simulink model "CM475A_TSG31CfgAndUse"  (R2013b)
settings: Solver=FixedStepDiscrete  SolverMode=SingleTasking  StartTime=0.0  StopTime=0.01  FixedStep=0.00005  RelTol=1e-3
values from neighbouring files (symbols this model uses):
  ELECGLBPRM_MOTCTRLINTRPTTRIGCFGB_CNT_U08 = DataDict.Constant    [CM475A_TSG31CfgAndUse_DataDict.m]
  ELECGLBPRM_MOTCTRLINTRPTTRIGSRC_CNT_U08 = DataDict.ConfigParam    [CM475A_TSG31CfgAndUse_DataDict.m]
  ELECGLBPRM_PWMPERDMIN_NANOSEC_U32 = DataDict.ConfigParam    [CM475A_TSG31CfgAndUse_DataDict.m]
  TSG31CfgAndUseAdcStrtOfCnvn2Offs = DataDict.Calibration    [CM475A_TSG31CfgAndUse_DataDict.m]
  TSG31CfgAndUseAdcStrtOfCnvnMotCtrlPeakOffs = DataDict.Calibration    [CM475A_TSG31CfgAndUse_DataDict.m]
  TSG31CfgAndUseAdcStrtOfCnvnMotCtrlVlyOffs = DataDict.Calibration    [CM475A_TSG31CfgAndUse_DataDict.m]
  TSG31CfgAndUseMtrAg0SPIStart = DataDict.Calibration    [CM475A_TSG31CfgAndUse_DataDict.m]
  TSG31CfgAndUsePwmDbnd = DataDict.Calibration    [CM475A_TSG31CfgAndUse_DataDict.m]
  TSG31UPD_NANOSEC_U32 = DataDict.Constant    [CM475A_TSG31CfgAndUse_DataDict.m]
undefined symbols (not defined in the file or in its folder): sigbuilder_block, SysSt1
libraries: simulink x11, CM475A_TSG31CfgAndUse_ModelLibrary_Rev001 x11
(part 3 of 5)

== system CM475A_TSG31CfgAndUse/TSG31CfgAndUse/TSG31CfgAndUsePer2/Transition to Enable/Map Pins to Peripheral/IoHwAb_SetFctPeriphPhaBLowrCmd ==
  CopyRight2 : Subsystem  Description=|  mask(Copyright Information){none=on}
      | Copyright info block.                                               
      |                                                                     
      | Place copyright information at the top of every subsystem in design.
      mask prompts: none "No parameters"
      mask help: Place copyright information at the top of every subsystem in design.
      mask Display:
      | NxtrConf = 'Nexteer Confidential';
      | 
      | sys = bdroot; %handle for the current model ("system")
      | first = get_param(sys,'Created');
      | first = first(end-3:end);  %year is last four digits
      | 
      | last = get_param(sys,'LastModifiedDate');
      | if isempty(last)
      |     last = datestr(now,'yyyy');
      | else
      |     last = last(end-3:end);
      | end
      | 
      | if strcmp(first,last)
      |     fprintf('%s -- Copyright %s Nexteer',NxtrConf,first)
      | else
      |     fprintf('%s -- %s%s- %s Nexteer',NxtrConf,char(169),first,last)
      | end

== system CM475A_TSG31CfgAndUse/TSG31CfgAndUse/TSG31CfgAndUsePer2/Transition to Enable/Map Pins to Peripheral/IoHwAb_SetFctPeriphPhaBUpprCmd ==
  CopyRight2 : Subsystem  Description=|  mask(Copyright Information){none=on}
      | Copyright info block.                                               
      |                                                                     
      | Place copyright information at the top of every subsystem in design.
      mask prompts: none "No parameters"
      mask help: Place copyright information at the top of every subsystem in design.
      mask Display:
      | NxtrConf = 'Nexteer Confidential';
      | 
      | sys = bdroot; %handle for the current model ("system")
      | first = get_param(sys,'Created');
      | first = first(end-3:end);  %year is last four digits
      | 
      | last = get_param(sys,'LastModifiedDate');
      | if isempty(last)
      |     last = datestr(now,'yyyy');
      | else
      |     last = last(end-3:end);
      | end
      | 
      | if strcmp(first,last)
      |     fprintf('%s -- Copyright %s Nexteer',NxtrConf,first)
      | else
      |     fprintf('%s -- %s%s- %s Nexteer',NxtrConf,char(169),first,last)
      | end

== system CM475A_TSG31CfgAndUse/TSG31CfgAndUse/TSG31CfgAndUsePer2/Transition to Enable/Map Pins to Peripheral/IoHwAb_SetFctPeriphPhaCLowrCmd ==
  CopyRight2 : Subsystem  Description=|  mask(Copyright Information){none=on}
      | Copyright info block.                                               
      |                                                                     
      | Place copyright information at the top of every subsystem in design.
      mask prompts: none "No parameters"
      mask help: Place copyright information at the top of every subsystem in design.
      mask Display:
      | NxtrConf = 'Nexteer Confidential';
      | 
      | sys = bdroot; %handle for the current model ("system")
      | first = get_param(sys,'Created');
      | first = first(end-3:end);  %year is last four digits
      | 
      | last = get_param(sys,'LastModifiedDate');
      | if isempty(last)
      |     last = datestr(now,'yyyy');
      | else
      |     last = last(end-3:end);
      | end
      | 
      | if strcmp(first,last)
      |     fprintf('%s -- Copyright %s Nexteer',NxtrConf,first)
      | else
      |     fprintf('%s -- %s%s- %s Nexteer',NxtrConf,char(169),first,last)
      | end

== system CM475A_TSG31CfgAndUse/TSG31CfgAndUse/TSG31CfgAndUsePer2/Transition to Enable/Map Pins to Peripheral/IoHwAb_SetFctPeriphPhaCUpprCmd ==
  CopyRight2 : Subsystem  Description=|  mask(Copyright Information){none=on}
      | Copyright info block.                                               
      |                                                                     
      | Place copyright information at the top of every subsystem in design.
      mask prompts: none "No parameters"
      mask help: Place copyright information at the top of every subsystem in design.
      mask Display:
      | NxtrConf = 'Nexteer Confidential';
      | 
      | sys = bdroot; %handle for the current model ("system")
      | first = get_param(sys,'Created');
      | first = first(end-3:end);  %year is last four digits
      | 
      | last = get_param(sys,'LastModifiedDate');
      | if isempty(last)
      |     last = datestr(now,'yyyy');
      | else
      |     last = last(end-3:end);
      | end
      | 
      | if strcmp(first,last)
      |     fprintf('%s -- Copyright %s Nexteer',NxtrConf,first)
      | else
      |     fprintf('%s -- %s%s- %s Nexteer',NxtrConf,char(169),first,last)
      | end

== system CM475A_TSG31CfgAndUse/TSG31CfgAndUse/TSG31CfgAndUseInit1/Determine TSG31CTL4/Determine TSG31PIE/Config - B/CopyRight2 ==

== system CM475A_TSG31CfgAndUse/TSG31CfgAndUse/TSG31CfgAndUseInit1/Determine TSG31CTL4/Determine TSG31PIE/Default Config/CopyRight2 ==

== system CM475A_TSG31CfgAndUse/TSG31CfgAndUse/TSG31CfgAndUseInit1/Map FET Ctrl Signals to GPIO and Set Low/Map Pins to GPIO/IoHwAb_SetFctGpioPhaALowrCmd/CopyRight2 ==

== system CM475A_TSG31CfgAndUse/TSG31CfgAndUse/TSG31CfgAndUseInit1/Map FET Ctrl Signals to GPIO and Set Low/Map Pins to GPIO/IoHwAb_SetFctGpioPhaAUpprCmd/CopyRight2 ==

== system CM475A_TSG31CfgAndUse/TSG31CfgAndUse/TSG31CfgAndUseInit1/Map FET Ctrl Signals to GPIO and Set Low/Map Pins to GPIO/IoHwAb_SetFctGpioPhaBLowrCmd/CopyRight2 ==

== system CM475A_TSG31CfgAndUse/TSG31CfgAndUse/TSG31CfgAndUseInit1/Map FET Ctrl Signals to GPIO and Set Low/Map Pins to GPIO/IoHwAb_SetFctGpioPhaBUpprCmd/CopyRight2 ==

== system CM475A_TSG31CfgAndUse/TSG31CfgAndUse/TSG31CfgAndUseInit1/Map FET Ctrl Signals to GPIO and Set Low/Map Pins to GPIO/IoHwAb_SetFctGpioPhaCLowrCmd/CopyRight2 ==

== system CM475A_TSG31CfgAndUse/TSG31CfgAndUse/TSG31CfgAndUseInit1/Map FET Ctrl Signals to GPIO and Set Low/Map Pins to GPIO/IoHwAb_SetFctGpioPhaCUpprCmd/CopyRight2 ==

== system CM475A_TSG31CfgAndUse/TSG31CfgAndUse/TSG31CfgAndUseInit1/Map FET Ctrl Signals to GPIO and Set Low/Set GPIO Level/IoHwAb_SetGpioPhaALowrCmd/CopyRight2 ==

== system CM475A_TSG31CfgAndUse/TSG31CfgAndUse/TSG31CfgAndUseInit1/Map FET Ctrl Signals to GPIO and Set Low/Set GPIO Level/IoHwAb_SetGpioPhaAUpprCmd/CopyRight2 ==

== system CM475A_TSG31CfgAndUse/TSG31CfgAndUse/TSG31CfgAndUseInit1/Map FET Ctrl Signals to GPIO and Set Low/Set GPIO Level/IoHwAb_SetGpioPhaBLowrCmd/CopyRight2 ==

== system CM475A_TSG31CfgAndUse/TSG31CfgAndUse/TSG31CfgAndUseInit1/Map FET Ctrl Signals to GPIO and Set Low/Set GPIO Level/IoHwAb_SetGpioPhaBUpprCmd/CopyRight2 ==

== system CM475A_TSG31CfgAndUse/TSG31CfgAndUse/TSG31CfgAndUseInit1/Map FET Ctrl Signals to GPIO and Set Low/Set GPIO Level/IoHwAb_SetGpioPhaCLowrCmd/CopyRight2 ==

== system CM475A_TSG31CfgAndUse/TSG31CfgAndUse/TSG31CfgAndUseInit1/Map FET Ctrl Signals to GPIO and Set Low/Set GPIO Level/IoHwAb_SetGpioPhaCUpprCmd/CopyRight2 ==

== system CM475A_TSG31CfgAndUse/TSG31CfgAndUse/TSG31CfgAndUsePer2/No Transition SysState = Enable/MCECS_CMDSAFEST/Map Pins to GPIO/CopyRight2 ==

== system CM475A_TSG31CfgAndUse/TSG31CfgAndUse/TSG31CfgAndUsePer2/No Transition SysState = Enable/MCECS_CMDSAFEST/Map Pins to GPIO/IoHwAb_SetFctGpioPhaALowrCmd ==
  CopyRight2 : Subsystem  Description=|  mask(Copyright Information){none=on}
      | Copyright info block.                                               
      |                                                                     
      | Place copyright information at the top of every subsystem in design.
      mask prompts: none "No parameters"
      mask help: Place copyright information at the top of every subsystem in design.
      mask Display:
      | NxtrConf = 'Nexteer Confidential';
      | 
      | sys = bdroot; %handle for the current model ("system")
      | first = get_param(sys,'Created');
      | first = first(end-3:end);  %year is last four digits
      | 
      | last = get_param(sys,'LastModifiedDate');
      | if isempty(last)
      |     last = datestr(now,'yyyy');
      | else
      |     last = last(end-3:end);
      | end
      | 
      | if strcmp(first,last)
      |     fprintf('%s -- Copyright %s Nexteer',NxtrConf,first)
      | else
      |     fprintf('%s -- %s%s- %s Nexteer',NxtrConf,char(169),first,last)
      | end

== system CM475A_TSG31CfgAndUse/TSG31CfgAndUse/TSG31CfgAndUsePer2/No Transition SysState = Enable/MCECS_CMDSAFEST/Map Pins to GPIO/IoHwAb_SetFctGpioPhaAUpprCmd ==
  CopyRight2 : Subsystem  Description=|  mask(Copyright Information){none=on}
      | Copyright info block.                                               
      |                                                                     
      | Place copyright information at the top of every subsystem in design.
      mask prompts: none "No parameters"
      mask help: Place copyright information at the top of every subsystem in design.
      mask Display:
      | NxtrConf = 'Nexteer Confidential';
      | 
      | sys = bdroot; %handle for the current model ("system")
      | first = get_param(sys,'Created');
      | first = first(end-3:end);  %year is last four digits
      | 
      | last = get_param(sys,'LastModifiedDate');
      | if isempty(last)
      |     last = datestr(now,'yyyy');
      | else
      |     last = last(end-3:end);
      | end
      | 
      | if strcmp(first,last)
      |     fprintf('%s -- Copyright %s Nexteer',NxtrConf,first)
      | else
      |     fprintf('%s -- %s%s- %s Nexteer',NxtrConf,char(169),first,last)
      | end

== system CM475A_TSG31CfgAndUse/TSG31CfgAndUse/TSG31CfgAndUsePer2/No Transition SysState = Enable/MCECS_CMDSAFEST/Map Pins to GPIO/IoHwAb_SetFctGpioPhaBLowrCmd ==
  CopyRight2 : Subsystem  Description=|  mask(Copyright Information){none=on}
      | Copyright info block.                                               
      |                                                                     
      | Place copyright information at the top of every subsystem in design.
      mask prompts: none "No parameters"
      mask help: Place copyright information at the top of every subsystem in design.
      mask Display:
      | NxtrConf = 'Nexteer Confidential';
      | 
      | sys = bdroot; %handle for the current model ("system")
      | first = get_param(sys,'Created');
      | first = first(end-3:end);  %year is last four digits
      | 
      | last = get_param(sys,'LastModifiedDate');
      | if isempty(last)
      |     last = datestr(now,'yyyy');
      | else
      |     last = last(end-3:end);
      | end
      | 
      | if strcmp(first,last)
      |     fprintf('%s -- Copyright %s Nexteer',NxtrConf,first)
      | else
      |     fprintf('%s -- %s%s- %s Nexteer',NxtrConf,char(169),first,last)
      | end

== system CM475A_TSG31CfgAndUse/TSG31CfgAndUse/TSG31CfgAndUsePer2/No Transition SysState = Enable/MCECS_CMDSAFEST/Map Pins to GPIO/IoHwAb_SetFctGpioPhaBUpprCmd ==
  CopyRight2 : Subsystem  Description=|  mask(Copyright Information){none=on}
      | Copyright info block.                                               
      |                                                                     
      | Place copyright information at the top of every subsystem in design.
      mask prompts: none "No parameters"
      mask help: Place copyright information at the top of every subsystem in design.
      mask Display:
      | NxtrConf = 'Nexteer Confidential';
      | 
      | sys = bdroot; %handle for the current model ("system")
      | first = get_param(sys,'Created');
      | first = first(end-3:end);  %year is last four digits
      | 
      | last = get_param(sys,'LastModifiedDate');
      | if isempty(last)
      |     last = datestr(now,'yyyy');
      | else
      |     last = last(end-3:end);
      | end
      | 
      | if strcmp(first,last)
      |     fprintf('%s -- Copyright %s Nexteer',NxtrConf,first)
      | else
      |     fprintf('%s -- %s%s- %s Nexteer',NxtrConf,char(169),first,last)
      | end

== system CM475A_TSG31CfgAndUse/TSG31CfgAndUse/TSG31CfgAndUsePer2/No Transition SysState = Enable/MCECS_CMDSAFEST/Map Pins to GPIO/IoHwAb_SetFctGpioPhaCLowrCmd ==
  CopyRight2 : Subsystem  Description=|  mask(Copyright Information){none=on}
      | Copyright info block.                                               
      |                                                                     
      | Place copyright information at the top of every subsystem in design.
      mask prompts: none "No parameters"
      mask help: Place copyright information at the top of every subsystem in design.
      mask Display:
      | NxtrConf = 'Nexteer Confidential';
      | 
      | sys = bdroot; %handle for the current model ("system")
      | first = get_param(sys,'Created');
      | first = first(end-3:end);  %year is last four digits
      | 
      | last = get_param(sys,'LastModifiedDate');
      | if isempty(last)
      |     last = datestr(now,'yyyy');
      | else
      |     last = last(end-3:end);
      | end
      | 
      | if strcmp(first,last)
      |     fprintf('%s -- Copyright %s Nexteer',NxtrConf,first)
      | else
      |     fprintf('%s -- %s%s- %s Nexteer',NxtrConf,char(169),first,last)
      | end

== system CM475A_TSG31CfgAndUse/TSG31CfgAndUse/TSG31CfgAndUsePer2/No Transition SysState = Enable/MCECS_CMDSAFEST/Map Pins to GPIO/IoHwAb_SetFctGpioPhaCUpprCmd ==
  CopyRight2 : Subsystem  Description=|  mask(Copyright Information){none=on}
      | Copyright info block.                                               
      |                                                                     
      | Place copyright information at the top of every subsystem in design.
      mask prompts: none "No parameters"
      mask help: Place copyright information at the top of every subsystem in design.
      mask Display:
      | NxtrConf = 'Nexteer Confidential';
      | 
      | sys = bdroot; %handle for the current model ("system")
      | first = get_param(sys,'Created');
      | first = first(end-3:end);  %year is last four digits
      | 
      | last = get_param(sys,'LastModifiedDate');
      | if isempty(last)
      |     last = datestr(now,'yyyy');
      | else
      |     last = last(end-3:end);
      | end
      | 
      | if strcmp(first,last)
      |     fprintf('%s -- Copyright %s Nexteer',NxtrConf,first)
      | else
      |     fprintf('%s -- %s%s- %s Nexteer',NxtrConf,char(169),first,last)
      | end

== system CM475A_TSG31CfgAndUse/TSG31CfgAndUse/TSG31CfgAndUsePer2/No Transition SysState = Enable/MCECS_CMDSAFEST/Set GPIO Level/CopyRight2 ==

== system CM475A_TSG31CfgAndUse/TSG31CfgAndUse/TSG31CfgAndUsePer2/No Transition SysState = Enable/MCECS_CMDSAFEST/Set GPIO Level/IoHwAb_SetGpioPhaALowrCmd ==
  PinSt : Inport  OutDataTypeStr=boolean
  CopyRight2 : Subsystem  Description=|  mask(Copyright Information){none=on}
      | Copyright info block.                                               
      |                                                                     
      | Place copyright information at the top of every subsystem in design.
      mask prompts: none "No parameters"
      mask help: Place copyright information at the top of every subsystem in design.
      mask Display:
      | NxtrConf = 'Nexteer Confidential';
      | 
      | sys = bdroot; %handle for the current model ("system")
      | first = get_param(sys,'Created');
      | first = first(end-3:end);  %year is last four digits
      | 
      | last = get_param(sys,'LastModifiedDate');
      | if isempty(last)
      |     last = datestr(now,'yyyy');
      | else
      |     last = last(end-3:end);
      | end
      | 
      | if strcmp(first,last)
      |     fprintf('%s -- Copyright %s Nexteer',NxtrConf,first)
      | else
      |     fprintf('%s -- %s%s- %s Nexteer',NxtrConf,char(169),first,last)
      | end
  Terminator : Terminator
  wires:
  PinSt/1 -> Terminator/1

== system CM475A_TSG31CfgAndUse/TSG31CfgAndUse/TSG31CfgAndUsePer2/No Transition SysState = Enable/MCECS_CMDSAFEST/Set GPIO Level/IoHwAb_SetGpioPhaAUpprCmd ==
  PinSt : Inport  OutDataTypeStr=boolean
  CopyRight2 : Subsystem  Description=|  mask(Copyright Information){none=on}
      | Copyright info block.                                               
      |                                                                     
      | Place copyright information at the top of every subsystem in design.
      mask prompts: none "No parameters"
      mask help: Place copyright information at the top of every subsystem in design.
      mask Display:
      | NxtrConf = 'Nexteer Confidential';
      | 
      | sys = bdroot; %handle for the current model ("system")
      | first = get_param(sys,'Created');
      | first = first(end-3:end);  %year is last four digits
      | 
      | last = get_param(sys,'LastModifiedDate');
      | if isempty(last)
      |     last = datestr(now,'yyyy');
      | else
      |     last = last(end-3:end);
      | end
      | 
      | if strcmp(first,last)
      |     fprintf('%s -- Copyright %s Nexteer',NxtrConf,first)
      | else
      |     fprintf('%s -- %s%s- %s Nexteer',NxtrConf,char(169),first,last)
      | end
  Terminator : Terminator
  wires:
  PinSt/1 -> Terminator/1

== system CM475A_TSG31CfgAndUse/TSG31CfgAndUse/TSG31CfgAndUsePer2/No Transition SysState = Enable/MCECS_CMDSAFEST/Set GPIO Level/IoHwAb_SetGpioPhaBLowrCmd ==
  PinSt : Inport  OutDataTypeStr=boolean
  CopyRight2 : Subsystem  Description=|  mask(Copyright Information){none=on}
      | Copyright info block.                                               
      |                                                                     
      | Place copyright information at the top of every subsystem in design.
      mask prompts: none "No parameters"
      mask help: Place copyright information at the top of every subsystem in design.
      mask Display:
      | NxtrConf = 'Nexteer Confidential';
      | 
      | sys = bdroot; %handle for the current model ("system")
      | first = get_param(sys,'Created');
      | first = first(end-3:end);  %year is last four digits
      | 
      | last = get_param(sys,'LastModifiedDate');
      | if isempty(last)
      |     last = datestr(now,'yyyy');
      | else
      |     last = last(end-3:end);
      | end
      | 
      | if strcmp(first,last)
      |     fprintf('%s -- Copyright %s Nexteer',NxtrConf,first)
      | else
      |     fprintf('%s -- %s%s- %s Nexteer',NxtrConf,char(169),first,last)
      | end
  Terminator : Terminator
  wires:
  PinSt/1 -> Terminator/1

== system CM475A_TSG31CfgAndUse/TSG31CfgAndUse/TSG31CfgAndUsePer2/No Transition SysState = Enable/MCECS_CMDSAFEST/Set GPIO Level/IoHwAb_SetGpioPhaBUpprCmd ==
  PinSt : Inport  OutDataTypeStr=boolean
  CopyRight2 : Subsystem  Description=|  mask(Copyright Information){none=on}
      | Copyright info block.                                               
      |                                                                     
      | Place copyright information at the top of every subsystem in design.
      mask prompts: none "No parameters"
      mask help: Place copyright information at the top of every subsystem in design.
      mask Display:
      | NxtrConf = 'Nexteer Confidential';
      | 
      | sys = bdroot; %handle for the current model ("system")
      | first = get_param(sys,'Created');
      | first = first(end-3:end);  %year is last four digits
      | 
      | last = get_param(sys,'LastModifiedDate');
      | if isempty(last)
      |     last = datestr(now,'yyyy');
      | else
      |     last = last(end-3:end);
      | end
      | 
      | if strcmp(first,last)
      |     fprintf('%s -- Copyright %s Nexteer',NxtrConf,first)
      | else
      |     fprintf('%s -- %s%s- %s Nexteer',NxtrConf,char(169),first,last)
      | end
  Terminator : Terminator
  wires:
  PinSt/1 -> Terminator/1

== system CM475A_TSG31CfgAndUse/TSG31CfgAndUse/TSG31CfgAndUsePer2/No Transition SysState = Enable/MCECS_CMDSAFEST/Set GPIO Level/IoHwAb_SetGpioPhaCLowrCmd ==
  PinSt : Inport  OutDataTypeStr=boolean
  CopyRight2 : Subsystem  Description=|  mask(Copyright Information){none=on}
      | Copyright info block.                                               
      |                                                                     
      | Place copyright information at the top of every subsystem in design.
      mask prompts: none "No parameters"
      mask help: Place copyright information at the top of every subsystem in design.
      mask Display:
      | NxtrConf = 'Nexteer Confidential';
      | 
      | sys = bdroot; %handle for the current model ("system")
      | first = get_param(sys,'Created');
      | first = first(end-3:end);  %year is last four digits
      | 
      | last = get_param(sys,'LastModifiedDate');
      | if isempty(last)
      |     last = datestr(now,'yyyy');
      | else
      |     last = last(end-3:end);
      | end
      | 
      | if strcmp(first,last)
      |     fprintf('%s -- Copyright %s Nexteer',NxtrConf,first)
      | else
      |     fprintf('%s -- %s%s- %s Nexteer',NxtrConf,char(169),first,last)
      | end
  Terminator : Terminator
  wires:
  PinSt/1 -> Terminator/1

== system CM475A_TSG31CfgAndUse/TSG31CfgAndUse/TSG31CfgAndUsePer2/No Transition SysState = Enable/MCECS_CMDSAFEST/Set GPIO Level/IoHwAb_SetGpioPhaCUpprCmd ==
  PinSt : Inport  OutDataTypeStr=boolean
  CopyRight2 : Subsystem  Description=|  mask(Copyright Information){none=on}
      | Copyright info block.                                               
      |                                                                     
      | Place copyright information at the top of every subsystem in design.
      mask prompts: none "No parameters"
      mask help: Place copyright information at the top of every subsystem in design.
      mask Display:
      | NxtrConf = 'Nexteer Confidential';
      | 
      | sys = bdroot; %handle for the current model ("system")
      | first = get_param(sys,'Created');
      | first = first(end-3:end);  %year is last four digits
      | 
      | last = get_param(sys,'LastModifiedDate');
      | if isempty(last)
      |     last = datestr(now,'yyyy');
      | else
      |     last = last(end-3:end);
      | end
      | 
      | if strcmp(first,last)
      |     fprintf('%s -- Copyright %s Nexteer',NxtrConf,first)
      | else
      |     fprintf('%s -- %s%s- %s Nexteer',NxtrConf,char(169),first,last)
      | end
  Terminator : Terminator
  wires:
  PinSt/1 -> Terminator/1

== system CM475A_TSG31CfgAndUse/TSG31CfgAndUse/TSG31CfgAndUsePer2/No Transition SysState = Enable/MCECS_GAINCMDBE/Map Pins to GPIO/CopyRight2 ==

== system CM475A_TSG31CfgAndUse/TSG31CfgAndUse/TSG31CfgAndUsePer2/No Transition SysState = Enable/MCECS_GAINCMDBE/Map Pins to GPIO/IoHwAb_SetFctGpioPhaALowrCmd ==
  CopyRight2 : Subsystem  Description=|  mask(Copyright Information){none=on}
      | Copyright info block.                                               
      |                                                                     
      | Place copyright information at the top of every subsystem in design.
      mask prompts: none "No parameters"
      mask help: Place copyright information at the top of every subsystem in design.
      mask Display:
      | NxtrConf = 'Nexteer Confidential';
      | 
      | sys = bdroot; %handle for the current model ("system")
      | first = get_param(sys,'Created');
      | first = first(end-3:end);  %year is last four digits
      | 
      | last = get_param(sys,'LastModifiedDate');
      | if isempty(last)
      |     last = datestr(now,'yyyy');
      | else
      |     last = last(end-3:end);
      | end
      | 
      | if strcmp(first,last)
      |     fprintf('%s -- Copyright %s Nexteer',NxtrConf,first)
      | else
      |     fprintf('%s -- %s%s- %s Nexteer',NxtrConf,char(169),first,last)
      | end

== system CM475A_TSG31CfgAndUse/TSG31CfgAndUse/TSG31CfgAndUsePer2/No Transition SysState = Enable/MCECS_GAINCMDBE/Map Pins to GPIO/IoHwAb_SetFctGpioPhaAUpprCmd ==
  CopyRight2 : Subsystem  Description=|  mask(Copyright Information){none=on}
      | Copyright info block.                                               
      |                                                                     
      | Place copyright information at the top of every subsystem in design.
      mask prompts: none "No parameters"
      mask help: Place copyright information at the top of every subsystem in design.
      mask Display:
      | NxtrConf = 'Nexteer Confidential';
      | 
      | sys = bdroot; %handle for the current model ("system")
      | first = get_param(sys,'Created');
      | first = first(end-3:end);  %year is last four digits
      | 
      | last = get_param(sys,'LastModifiedDate');
      | if isempty(last)
      |     last = datestr(now,'yyyy');
      | else
      |     last = last(end-3:end);
      | end
      | 
      | if strcmp(first,last)
      |     fprintf('%s -- Copyright %s Nexteer',NxtrConf,first)
      | else
      |     fprintf('%s -- %s%s- %s Nexteer',NxtrConf,char(169),first,last)
      | end

== system CM475A_TSG31CfgAndUse/TSG31CfgAndUse/TSG31CfgAndUsePer2/No Transition SysState = Enable/MCECS_GAINCMDBE/Map Pins to GPIO/IoHwAb_SetFctGpioPhaBLowrCmd ==
  CopyRight2 : Subsystem  Description=|  mask(Copyright Information){none=on}
      | Copyright info block.                                               
      |                                                                     
      | Place copyright information at the top of every subsystem in design.
      mask prompts: none "No parameters"
      mask help: Place copyright information at the top of every subsystem in design.
      mask Display:
      | NxtrConf = 'Nexteer Confidential';
      | 
      | sys = bdroot; %handle for the current model ("system")
      | first = get_param(sys,'Created');
      | first = first(end-3:end);  %year is last four digits
      | 
      | last = get_param(sys,'LastModifiedDate');
      | if isempty(last)
      |     last = datestr(now,'yyyy');
      | else
      |     last = last(end-3:end);
      | end
      | 
      | if strcmp(first,last)
      |     fprintf('%s -- Copyright %s Nexteer',NxtrConf,first)
      | else
      |     fprintf('%s -- %s%s- %s Nexteer',NxtrConf,char(169),first,last)
      | end

== system CM475A_TSG31CfgAndUse/TSG31CfgAndUse/TSG31CfgAndUsePer2/No Transition SysState = Enable/MCECS_GAINCMDBE/Map Pins to GPIO/IoHwAb_SetFctGpioPhaBUpprCmd ==
  CopyRight2 : Subsystem  Description=|  mask(Copyright Information){none=on}
      | Copyright info block.                                               
      |                                                                     
      | Place copyright information at the top of every subsystem in design.
      mask prompts: none "No parameters"
      mask help: Place copyright information at the top of every subsystem in design.
      mask Display:
      | NxtrConf = 'Nexteer Confidential';
      | 
      | sys = bdroot; %handle for the current model ("system")
      | first = get_param(sys,'Created');
      | first = first(end-3:end);  %year is last four digits
      | 
      | last = get_param(sys,'LastModifiedDate');
      | if isempty(last)
      |     last = datestr(now,'yyyy');
      | else
      |     last = last(end-3:end);
      | end
      | 
      | if strcmp(first,last)
      |     fprintf('%s -- Copyright %s Nexteer',NxtrConf,first)
      | else
      |     fprintf('%s -- %s%s- %s Nexteer',NxtrConf,char(169),first,last)
      | end

== system CM475A_TSG31CfgAndUse/TSG31CfgAndUse/TSG31CfgAndUsePer2/No Transition SysState = Enable/MCECS_GAINCMDBE/Map Pins to GPIO/IoHwAb_SetFctGpioPhaCLowrCmd ==
  CopyRight2 : Subsystem  Description=|  mask(Copyright Information){none=on}
      | Copyright info block.                                               
      |                                                                     
      | Place copyright information at the top of every subsystem in design.
      mask prompts: none "No parameters"
      mask help: Place copyright information at the top of every subsystem in design.
      mask Display:
      | NxtrConf = 'Nexteer Confidential';
      | 
      | sys = bdroot; %handle for the current model ("system")
      | first = get_param(sys,'Created');
      | first = first(end-3:end);  %year is last four digits
      | 
      | last = get_param(sys,'LastModifiedDate');
      | if isempty(last)
      |     last = datestr(now,'yyyy');
      | else
      |     last = last(end-3:end);
      | end
      | 
      | if strcmp(first,last)
      |     fprintf('%s -- Copyright %s Nexteer',NxtrConf,first)
      | else
      |     fprintf('%s -- %s%s- %s Nexteer',NxtrConf,char(169),first,last)
      | end

== system CM475A_TSG31CfgAndUse/TSG31CfgAndUse/TSG31CfgAndUsePer2/No Transition SysState = Enable/MCECS_GAINCMDBE/Map Pins to GPIO/IoHwAb_SetFctGpioPhaCUpprCmd ==
  CopyRight2 : Subsystem  Description=|  mask(Copyright Information){none=on}
      | Copyright info block.                                               
      |                                                                     
      | Place copyright information at the top of every subsystem in design.
      mask prompts: none "No parameters"
      mask help: Place copyright information at the top of every subsystem in design.
      mask Display:
      | NxtrConf = 'Nexteer Confidential';
      | 
      | sys = bdroot; %handle for the current model ("system")
      | first = get_param(sys,'Created');
      | first = first(end-3:end);  %year is last four digits
      | 
      | last = get_param(sys,'LastModifiedDate');
      | if isempty(last)
      |     last = datestr(now,'yyyy');
      | else
      |     last = last(end-3:end);
      | end
      | 
      | if strcmp(first,last)
      |     fprintf('%s -- Copyright %s Nexteer',NxtrConf,first)
      | else
      |     fprintf('%s -- %s%s- %s Nexteer',NxtrConf,char(169),first,last)
      | end

== system CM475A_TSG31CfgAndUse/TSG31CfgAndUse/TSG31CfgAndUsePer2/No Transition SysState = Enable/MCECS_GAINCMDBE/Set GPIO Level/CopyRight2 ==

== system CM475A_TSG31CfgAndUse/TSG31CfgAndUse/TSG31CfgAndUsePer2/No Transition SysState = Enable/MCECS_GAINCMDBE/Set GPIO Level/IoHwAb_SetGpioPhaALowrCmd ==
  PinSt : Inport  OutDataTypeStr=boolean
  CopyRight2 : Subsystem  Description=|  mask(Copyright Information){none=on}
      | Copyright info block.                                               
      |                                                                     
      | Place copyright information at the top of every subsystem in design.
      mask prompts: none "No parameters"
      mask help: Place copyright information at the top of every subsystem in design.
      mask Display:
      | NxtrConf = 'Nexteer Confidential';
      | 
      | sys = bdroot; %handle for the current model ("system")
      | first = get_param(sys,'Created');
      | first = first(end-3:end);  %year is last four digits
      | 
      | last = get_param(sys,'LastModifiedDate');
      | if isempty(last)
      |     last = datestr(now,'yyyy');
      | else
      |     last = last(end-3:end);
      | end
      | 
      | if strcmp(first,last)
      |     fprintf('%s -- Copyright %s Nexteer',NxtrConf,first)
      | else
      |     fprintf('%s -- %s%s- %s Nexteer',NxtrConf,char(169),first,last)
      | end
  Terminator : Terminator
  wires:
  PinSt/1 -> Terminator/1

== system CM475A_TSG31CfgAndUse/TSG31CfgAndUse/TSG31CfgAndUsePer2/No Transition SysState = Enable/MCECS_GAINCMDBE/Set GPIO Level/IoHwAb_SetGpioPhaAUpprCmd ==
  PinSt : Inport  OutDataTypeStr=boolean
  CopyRight2 : Subsystem  Description=|  mask(Copyright Information){none=on}
      | Copyright info block.                                               
      |                                                                     
      | Place copyright information at the top of every subsystem in design.
      mask prompts: none "No parameters"
      mask help: Place copyright information at the top of every subsystem in design.
      mask Display:
      | NxtrConf = 'Nexteer Confidential';
      | 
      | sys = bdroot; %handle for the current model ("system")
      | first = get_param(sys,'Created');
      | first = first(end-3:end);  %year is last four digits
      | 
      | last = get_param(sys,'LastModifiedDate');
      | if isempty(last)
      |     last = datestr(now,'yyyy');
      | else
      |     last = last(end-3:end);
      | end
      | 
      | if strcmp(first,last)
      |     fprintf('%s -- Copyright %s Nexteer',NxtrConf,first)
      | else
      |     fprintf('%s -- %s%s- %s Nexteer',NxtrConf,char(169),first,last)
      | end
  Terminator : Terminator
  wires:
  PinSt/1 -> Terminator/1

== system CM475A_TSG31CfgAndUse/TSG31CfgAndUse/TSG31CfgAndUsePer2/No Transition SysState = Enable/MCECS_GAINCMDBE/Set GPIO Level/IoHwAb_SetGpioPhaBLowrCmd ==
  PinSt : Inport  OutDataTypeStr=boolean
  CopyRight2 : Subsystem  Description=|  mask(Copyright Information){none=on}
      | Copyright info block.                                               
      |                                                                     
      | Place copyright information at the top of every subsystem in design.
      mask prompts: none "No parameters"
      mask help: Place copyright information at the top of every subsystem in design.
      mask Display:
      | NxtrConf = 'Nexteer Confidential';
      | 
      | sys = bdroot; %handle for the current model ("system")
      | first = get_param(sys,'Created');
      | first = first(end-3:end);  %year is last four digits
      | 
      | last = get_param(sys,'LastModifiedDate');
      | if isempty(last)
      |     last = datestr(now,'yyyy');
      | else
      |     last = last(end-3:end);
      | end
      | 
      | if strcmp(first,last)
      |     fprintf('%s -- Copyright %s Nexteer',NxtrConf,first)
      | else
      |     fprintf('%s -- %s%s- %s Nexteer',NxtrConf,char(169),first,last)
      | end
  Terminator : Terminator
  wires:
  PinSt/1 -> Terminator/1

== system CM475A_TSG31CfgAndUse/TSG31CfgAndUse/TSG31CfgAndUsePer2/No Transition SysState = Enable/MCECS_GAINCMDBE/Set GPIO Level/IoHwAb_SetGpioPhaBUpprCmd ==
  PinSt : Inport  OutDataTypeStr=boolean
  CopyRight2 : Subsystem  Description=|  mask(Copyright Information){none=on}
      | Copyright info block.                                               
      |                                                                     
      | Place copyright information at the top of every subsystem in design.
      mask prompts: none "No parameters"
      mask help: Place copyright information at the top of every subsystem in design.
      mask Display:
      | NxtrConf = 'Nexteer Confidential';
      | 
      | sys = bdroot; %handle for the current model ("system")
      | first = get_param(sys,'Created');
      | first = first(end-3:end);  %year is last four digits
      | 
      | last = get_param(sys,'LastModifiedDate');
      | if isempty(last)
      |     last = datestr(now,'yyyy');
      | else
      |     last = last(end-3:end);
      | end
      | 
      | if strcmp(first,last)
      |     fprintf('%s -- Copyright %s Nexteer',NxtrConf,first)
      | else
      |     fprintf('%s -- %s%s- %s Nexteer',NxtrConf,char(169),first,last)
      | end
  Terminator : Terminator
  wires:
  PinSt/1 -> Terminator/1

== system CM475A_TSG31CfgAndUse/TSG31CfgAndUse/TSG31CfgAndUsePer2/No Transition SysState = Enable/MCECS_GAINCMDBE/Set GPIO Level/IoHwAb_SetGpioPhaCLowrCmd ==
  PinSt : Inport  OutDataTypeStr=boolean
  CopyRight2 : Subsystem  Description=|  mask(Copyright Information){none=on}
      | Copyright info block.                                               
      |                                                                     
      | Place copyright information at the top of every subsystem in design.
      mask prompts: none "No parameters"
      mask help: Place copyright information at the top of every subsystem in design.
      mask Display:
      | NxtrConf = 'Nexteer Confidential';
      | 
      | sys = bdroot; %handle for the current model ("system")
      | first = get_param(sys,'Created');
      | first = first(end-3:end);  %year is last four digits
      | 
      | last = get_param(sys,'LastModifiedDate');
      | if isempty(last)
      |     last = datestr(now,'yyyy');
      | else
      |     last = last(end-3:end);
      | end
      | 
      | if strcmp(first,last)
      |     fprintf('%s -- Copyright %s Nexteer',NxtrConf,first)
      | else
      |     fprintf('%s -- %s%s- %s Nexteer',NxtrConf,char(169),first,last)
      | end
  Terminator : Terminator
  wires:
  PinSt/1 -> Terminator/1

== system CM475A_TSG31CfgAndUse/TSG31CfgAndUse/TSG31CfgAndUsePer2/No Transition SysState = Enable/MCECS_GAINCMDBE/Set GPIO Level/IoHwAb_SetGpioPhaCUpprCmd ==
  PinSt : Inport  OutDataTypeStr=boolean
  CopyRight2 : Subsystem  Description=|  mask(Copyright Information){none=on}
      | Copyright info block.                                               
      |                                                                     
      | Place copyright information at the top of every subsystem in design.
      mask prompts: none "No parameters"
      mask help: Place copyright information at the top of every subsystem in design.
      mask Display:
      | NxtrConf = 'Nexteer Confidential';
      | 
      | sys = bdroot; %handle for the current model ("system")
      | first = get_param(sys,'Created');
      | first = first(end-3:end);  %year is last four digits
      | 
      | last = get_param(sys,'LastModifiedDate');
      | if isempty(last)
      |     last = datestr(now,'yyyy');
      | else
      |     last = last(end-3:end);
      | end
      | 
      | if strcmp(first,last)
      |     fprintf('%s -- Copyright %s Nexteer',NxtrConf,first)
      | else
      |     fprintf('%s -- %s%s- %s Nexteer',NxtrConf,char(169),first,last)
      | end
  Terminator : Terminator
  wires:
  PinSt/1 -> Terminator/1

== system CM475A_TSG31CfgAndUse/TSG31CfgAndUse/TSG31CfgAndUsePer2/No Transition SysState = Enable/MCECS_GAINCMDCF/Map Pins to GPIO/CopyRight2 ==

== system CM475A_TSG31CfgAndUse/TSG31CfgAndUse/TSG31CfgAndUsePer2/No Transition SysState = Enable/MCECS_GAINCMDCF/Map Pins to GPIO/IoHwAb_SetFctGpioPhaALowrCmd ==
  CopyRight2 : Subsystem  Description=|  mask(Copyright Information){none=on}
      | Copyright info block.                                               
      |                                                                     
      | Place copyright information at the top of every subsystem in design.
      mask prompts: none "No parameters"
      mask help: Place copyright information at the top of every subsystem in design.
      mask Display:
      | NxtrConf = 'Nexteer Confidential';
      | 
      | sys = bdroot; %handle for the current model ("system")
      | first = get_param(sys,'Created');
      | first = first(end-3:end);  %year is last four digits
      | 
      | last = get_param(sys,'LastModifiedDate');
      | if isempty(last)
      |     last = datestr(now,'yyyy');
      | else
      |     last = last(end-3:end);
      | end
      | 
      | if strcmp(first,last)
      |     fprintf('%s -- Copyright %s Nexteer',NxtrConf,first)
      | else
      |     fprintf('%s -- %s%s- %s Nexteer',NxtrConf,char(169),first,last)
      | end

== system CM475A_TSG31CfgAndUse/TSG31CfgAndUse/TSG31CfgAndUsePer2/No Transition SysState = Enable/MCECS_GAINCMDCF/Map Pins to GPIO/IoHwAb_SetFctGpioPhaAUpprCmd ==
  CopyRight2 : Subsystem  Description=|  mask(Copyright Information){none=on}
      | Copyright info block.                                               
      |                                                                     
      | Place copyright information at the top of every subsystem in design.
      mask prompts: none "No parameters"
      mask help: Place copyright information at the top of every subsystem in design.
      mask Display:
      | NxtrConf = 'Nexteer Confidential';
      | 
      | sys = bdroot; %handle for the current model ("system")
      | first = get_param(sys,'Created');
      | first = first(end-3:end);  %year is last four digits
      | 
      | last = get_param(sys,'LastModifiedDate');
      | if isempty(last)
      |     last = datestr(now,'yyyy');
      | else
      |     last = last(end-3:end);
      | end
      | 
      | if strcmp(first,last)
      |     fprintf('%s -- Copyright %s Nexteer',NxtrConf,first)
      | else
      |     fprintf('%s -- %s%s- %s Nexteer',NxtrConf,char(169),first,last)
      | end

== system CM475A_TSG31CfgAndUse/TSG31CfgAndUse/TSG31CfgAndUsePer2/No Transition SysState = Enable/MCECS_GAINCMDCF/Map Pins to GPIO/IoHwAb_SetFctGpioPhaBLowrCmd ==
  CopyRight2 : Subsystem  Description=|  mask(Copyright Information){none=on}
      | Copyright info block.                                               
      |                                                                     
      | Place copyright information at the top of every subsystem in design.
      mask prompts: none "No parameters"
      mask help: Place copyright information at the top of every subsystem in design.
      mask Display:
      | NxtrConf = 'Nexteer Confidential';
      | 
      | sys = bdroot; %handle for the current model ("system")
      | first = get_param(sys,'Created');
      | first = first(end-3:end);  %year is last four digits
      | 
      | last = get_param(sys,'LastModifiedDate');
      | if isempty(last)
      |     last = datestr(now,'yyyy');
      | else
      |     last = last(end-3:end);
      | end
      | 
      | if strcmp(first,last)
      |     fprintf('%s -- Copyright %s Nexteer',NxtrConf,first)
      | else
      |     fprintf('%s -- %s%s- %s Nexteer',NxtrConf,char(169),first,last)
      | end

== system CM475A_TSG31CfgAndUse/TSG31CfgAndUse/TSG31CfgAndUsePer2/No Transition SysState = Enable/MCECS_GAINCMDCF/Map Pins to GPIO/IoHwAb_SetFctGpioPhaBUpprCmd ==
  CopyRight2 : Subsystem  Description=|  mask(Copyright Information){none=on}
      | Copyright info block.                                               
      |                                                                     
      | Place copyright information at the top of every subsystem in design.
      mask prompts: none "No parameters"
      mask help: Place copyright information at the top of every subsystem in design.
      mask Display:
      | NxtrConf = 'Nexteer Confidential';
      | 
      | sys = bdroot; %handle for the current model ("system")
      | first = get_param(sys,'Created');
      | first = first(end-3:end);  %year is last four digits
      | 
      | last = get_param(sys,'LastModifiedDate');
      | if isempty(last)
      |     last = datestr(now,'yyyy');
      | else
      |     last = last(end-3:end);
      | end
      | 
      | if strcmp(first,last)
      |     fprintf('%s -- Copyright %s Nexteer',NxtrConf,first)
      | else
      |     fprintf('%s -- %s%s- %s Nexteer',NxtrConf,char(169),first,last)
      | end

== system CM475A_TSG31CfgAndUse/TSG31CfgAndUse/TSG31CfgAndUsePer2/No Transition SysState = Enable/MCECS_GAINCMDCF/Map Pins to GPIO/IoHwAb_SetFctGpioPhaCLowrCmd ==
  CopyRight2 : Subsystem  Description=|  mask(Copyright Information){none=on}
      | Copyright info block.                                               
      |                                                                     
      | Place copyright information at the top of every subsystem in design.
      mask prompts: none "No parameters"
      mask help: Place copyright information at the top of every subsystem in design.
      mask Display:
      | NxtrConf = 'Nexteer Confidential';
      | 
      | sys = bdroot; %handle for the current model ("system")
      | first = get_param(sys,'Created');
      | first = first(end-3:end);  %year is last four digits
      | 
      | last = get_param(sys,'LastModifiedDate');
      | if isempty(last)
      |     last = datestr(now,'yyyy');
      | else
      |     last = last(end-3:end);
      | end
      | 
      | if strcmp(first,last)
      |     fprintf('%s -- Copyright %s Nexteer',NxtrConf,first)
      | else
      |     fprintf('%s -- %s%s- %s Nexteer',NxtrConf,char(169),first,last)
      | end

== system CM475A_TSG31CfgAndUse/TSG31CfgAndUse/TSG31CfgAndUsePer2/No Transition SysState = Enable/MCECS_GAINCMDCF/Map Pins to GPIO/IoHwAb_SetFctGpioPhaCUpprCmd ==
  CopyRight2 : Subsystem  Description=|  mask(Copyright Information){none=on}
      | Copyright info block.                                               
      |                                                                     
      | Place copyright information at the top of every subsystem in design.
      mask prompts: none "No parameters"
      mask help: Place copyright information at the top of every subsystem in design.
      mask Display:
      | NxtrConf = 'Nexteer Confidential';
      | 
      | sys = bdroot; %handle for the current model ("system")
      | first = get_param(sys,'Created');
      | first = first(end-3:end);  %year is last four digits
      | 
      | last = get_param(sys,'LastModifiedDate');
      | if isempty(last)
      |     last = datestr(now,'yyyy');
      | else
      |     last = last(end-3:end);
      | end
      | 
      | if strcmp(first,last)
      |     fprintf('%s -- Copyright %s Nexteer',NxtrConf,first)
      | else
      |     fprintf('%s -- %s%s- %s Nexteer',NxtrConf,char(169),first,last)
      | end

== system CM475A_TSG31CfgAndUse/TSG31CfgAndUse/TSG31CfgAndUsePer2/No Transition SysState = Enable/MCECS_GAINCMDCF/Set GPIO Level/CopyRight2 ==

== system CM475A_TSG31CfgAndUse/TSG31CfgAndUse/TSG31CfgAndUsePer2/No Transition SysState = Enable/MCECS_GAINCMDCF/Set GPIO Level/IoHwAb_SetGpioPhaALowrCmd ==
  PinSt : Inport  OutDataTypeStr=boolean
  CopyRight2 : Subsystem  Description=|  mask(Copyright Information){none=on}
      | Copyright info block.                                               
      |                                                                     
      | Place copyright information at the top of every subsystem in design.
      mask prompts: none "No parameters"
      mask help: Place copyright information at the top of every subsystem in design.
      mask Display:
      | NxtrConf = 'Nexteer Confidential';
      | 
      | sys = bdroot; %handle for the current model ("system")
      | first = get_param(sys,'Created');
      | first = first(end-3:end);  %year is last four digits
      | 
      | last = get_param(sys,'LastModifiedDate');
      | if isempty(last)
      |     last = datestr(now,'yyyy');
      | else
      |     last = last(end-3:end);
      | end
      | 
      | if strcmp(first,last)
      |     fprintf('%s -- Copyright %s Nexteer',NxtrConf,first)
      | else
      |     fprintf('%s -- %s%s- %s Nexteer',NxtrConf,char(169),first,last)
      | end
  Terminator : Terminator
  wires:
  PinSt/1 -> Terminator/1

== system CM475A_TSG31CfgAndUse/TSG31CfgAndUse/TSG31CfgAndUsePer2/No Transition SysState = Enable/MCECS_GAINCMDCF/Set GPIO Level/IoHwAb_SetGpioPhaAUpprCmd ==
  PinSt : Inport  OutDataTypeStr=boolean
  CopyRight2 : Subsystem  Description=|  mask(Copyright Information){none=on}
      | Copyright info block.                                               
      |                                                                     
      | Place copyright information at the top of every subsystem in design.
      mask prompts: none "No parameters"
      mask help: Place copyright information at the top of every subsystem in design.
      mask Display:
      | NxtrConf = 'Nexteer Confidential';
      | 
      | sys = bdroot; %handle for the current model ("system")
      | first = get_param(sys,'Created');
      | first = first(end-3:end);  %year is last four digits
      | 
      | last = get_param(sys,'LastModifiedDate');
      | if isempty(last)
      |     last = datestr(now,'yyyy');
      | else
      |     last = last(end-3:end);
      | end
      | 
      | if strcmp(first,last)
      |     fprintf('%s -- Copyright %s Nexteer',NxtrConf,first)
      | else
      |     fprintf('%s -- %s%s- %s Nexteer',NxtrConf,char(169),first,last)
      | end
  Terminator : Terminator
  wires:
  PinSt/1 -> Terminator/1
